simulink model "twoareajai"  (Simulink 7.3)
settings: Solver=ode45  StartTime=0.0  StopTime=50  RelTol=1e-3
libraries: powerlib x1
settings Model: Creator=jeyashree  LastModifiedBy=Twad1

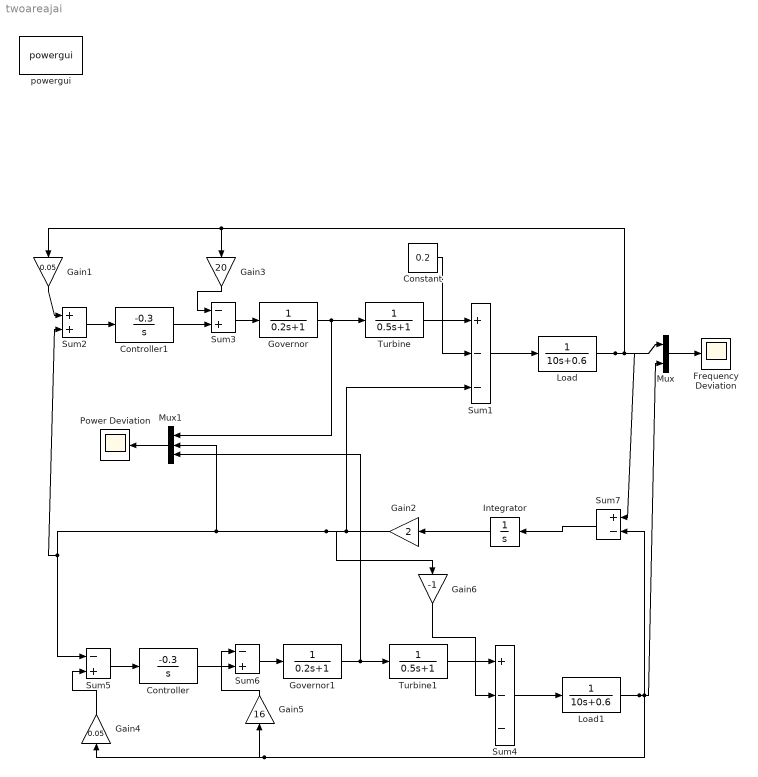
== system twoareajai ==
  Constant : Constant  Value=0.2  OutDataType=fixdt(1, 16)  OutScaling=2^0
  Controller : TransferFcn  Numerator=[-0.3]  Denominator=[1 0]
  Controller1 : TransferFcn  Numerator=[-0.3]  Denominator=[1 0]
  Frequency Deviation : Scope
      settings: TickLabels=on  SaveName=Frequency
  Gain1 : Gain  Gain=0.05
  Gain2 : Gain  Gain=2
  Gain3 : Gain  Gain=20
  Gain4 : Gain  Gain=0.05
  Gain5 : Gain  Gain=16
  Gain6 : Gain  Gain=-1
  Governor : TransferFcn  Denominator=[0.2 1]
  Governor1 : TransferFcn  Denominator=[0.2 1]
  Integrator : Integrator
  Load : TransferFcn  Denominator=[10 0.6]
  Load1 : TransferFcn  Denominator=[10 0.6]
  Mux : Mux  Inputs=2
  Mux1 : Mux  Inputs=3
  Power Deviation : Scope
      settings: SaveName=power  DataFormat=Array
  Sum1 : Sum  Inputs=+--
  Sum2 : Sum
  Sum3 : Sum  Inputs=-+
  Sum4 : Sum  Inputs=+--
  Sum5 : Sum  Inputs=-+
  Sum6 : Sum  Inputs=-+
  Sum7 : Sum  Inputs=+-
  Turbine : TransferFcn  Denominator=[0.5 1]
  Turbine1 : TransferFcn  Denominator=[0.5 1]
  powergui : powerlib/powergui  Priority=1  SystemSampleTime=-1  SimulationMode=Continuous  SampleTime=50e-6  frequency=60  SPID=off  DisableSnubberDevices=off  DisableRonSwitches=off  DisableVfSwitches=off  SwTol=0  Interpol=off  frequencyindice=60  echomessages=off  HookPort=off  DisplayEquations=off  FunctionMessages=off  EnableUseOfTLC=off  x0status=blocks  RestoreLinks=warning  Frange=[0:2:500]  Ylog=off  Xlog=on  ShowGrid=off  save=off  variable=ZData  structure=0  ZoomFFT=off  StartTime=0.0  cycles=1  DisplayStyle=1  fundamental=60  FreqAxis=off  MaxFrequency=1000  frequencyindicesteady=1  RmsSteady=1  display=off  Ts=100  methode=off
  wires:
  Sum1/1 -> Load/1
  Integrator/1 -> Gain2/1
  Sum2/1 -> Controller1/1
  Gain1/1 -> Sum2/1
  Controller1/1 -> Sum3/2
  Gain3/1 -> Sum3/1
  Sum3/1 -> Governor/1
  Governor/1 -> Turbine/1, Mux1/1
  Turbine/1 -> Sum1/1
  Constant/1 -> Sum1/2
  Load/1 -> Mux/1, Sum7/1, Gain1/1, Gain3/1
  Mux/1 -> Frequency Deviation/1
  Sum4/1 -> Load1/1
  Sum5/1 -> Controller/1
  Controller/1 -> Sum6/2
  Gain5/1 -> Sum6/1
  Sum6/1 -> Governor1/1
  Governor1/1 -> Turbine1/1, Mux1/3
  Turbine1/1 -> Sum4/1
  Load1/1 -> Sum7/2, Gain4/1, Gain5/1, Mux/2
  Gain4/1 -> Sum5/2
  Gain2/1 -> Gain6/1, Sum5/1, Sum2/2, Mux1/2, Sum1/3
  Gain6/1 -> Sum4/2
  Sum7/1 -> Integrator/1
  Mux1/1 -> Power Deviation/1
